simulink model "Fuel_slosh_practice"  (R2022b)
settings: Solver=FixedStepAuto  StartTime=0.0  StopTime=50.0  FixedStep=1e-3  RelTol=1e-3
values from neighbouring files (symbols this model uses):
  b = 0.1    [param.m]
  d1 = 6    [param.m]
  d2 = 10    [param.m]
  g = 9.80665    [sloshParams.m]
  k = 0.1    [param.m]
  k1 = 3    [param.m]
  k2 = 5    [param.m]
  m = 1    [param.m]
  m1 = 2    [param.m]
  m2 = 2    [param.m]
undefined symbols (not defined in the file or in its folder): L1, L2, theta1_0, theta2_0
settings Model: Creator=Aras Güngöre  LastModifiedBy=trameshk
settings SolverCC: AlgebraicLoopSolver=TrustRegion
settings DebuggingCC: UnconnectedInputMsg=warning  UnconnectedOutputMsg=warning  UnconnectedLineMsg=warning  SFMachineParentedDataDiag=warning
settings ModelReferenceCC: EnableRefExpFcnMdlSchedulingChecks=on
settings RTWCC: DLArmComputeVersion=19.05

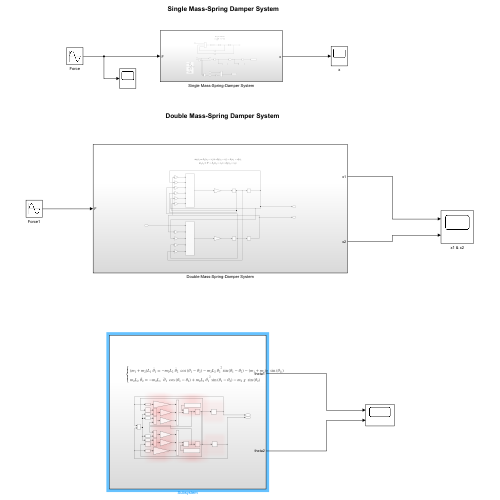
[thumbnail: Simulink's stored preview of the top-level diagram]
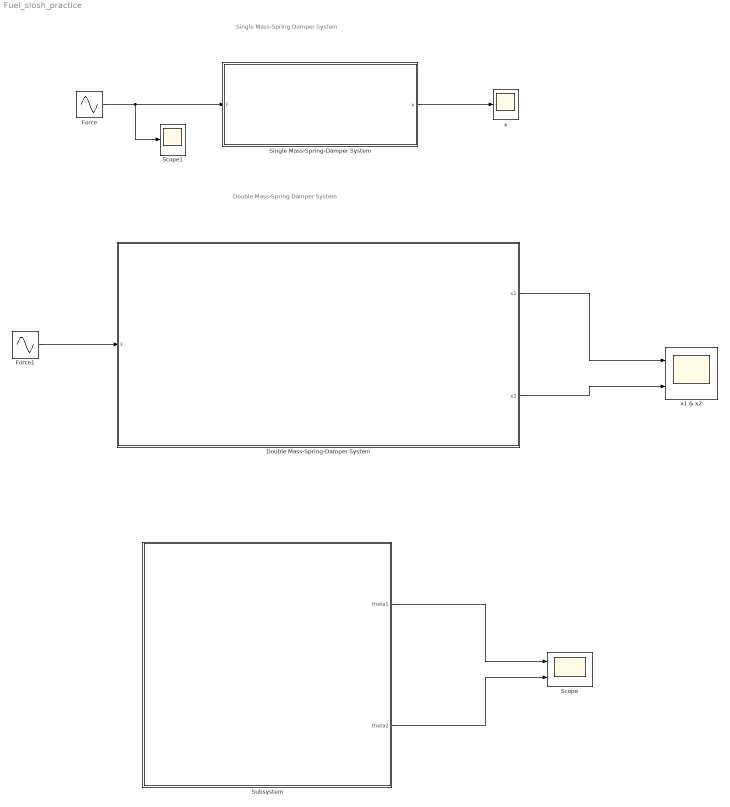
== system Fuel_slosh_practice ==
  note: Single Mass-Spring Damper System
  note: Double Mass-Spring Damper System
  Double Mass-Spring-Damper System : Subsystem
  Force : Sin  SampleTime=0
  Force1 : Sin  SampleTime=0
  Scope : Scope  NumInputPorts=2
  Scope1 : Scope
  Single Mass-Spring-Damper System : Subsystem
  Subsystem : Subsystem
  x : Scope
  x1 & x2 : Scope  NumInputPorts=2
  wires:
  Force/1 -> Scope1/1, Single Mass-Spring-Damper System/1(F)
  Single Mass-Spring-Damper System/1(x) -> x/1
  Force1/1 -> Double Mass-Spring-Damper System/1(F)
  Double Mass-Spring-Damper System/1(x1) -> x1 & x2/1
  Double Mass-Spring-Damper System/2(x2) -> x1 & x2/2
  Subsystem/2(theta2) -> Scope/2
  Subsystem/1(theta1) -> Scope/1

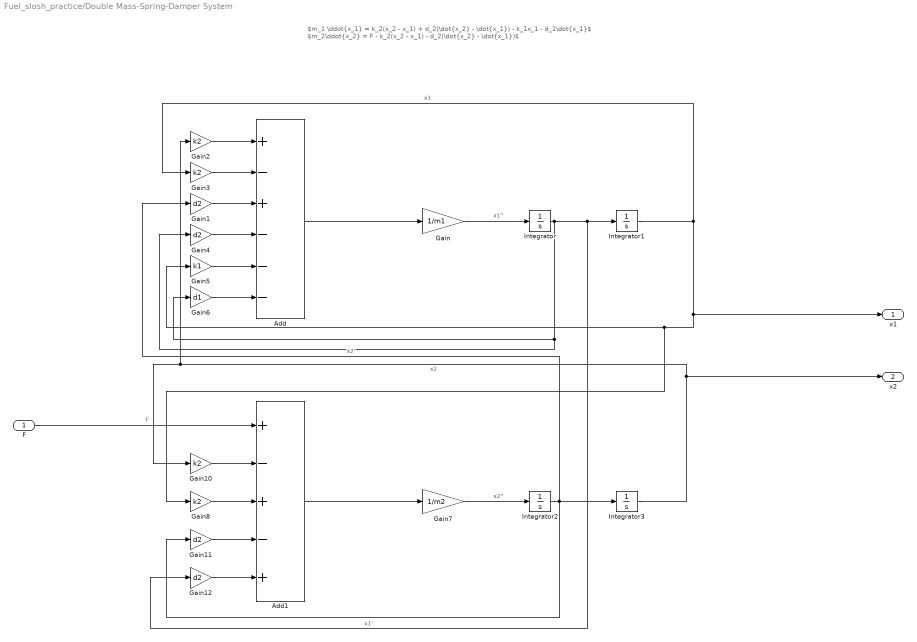
== system Fuel_slosh_practice/Double Mass-Spring-Damper System ==
  note: $m_1 \ddot{x_1} = k_2(x_2 - x_1) + d_2(\dot{x_2} - \dot{x_1}) - k_1x_1 - d_1\dot{x_1}$ $m_2\ddot{x_2} = F - k_2(x_2 - x_1) - d_2(\dot{x_2} - \dot{x_1})$
  F : Inport
  Add : Sum  Inputs=+-+---
  Add1 : Sum  Inputs=+-+-+
  Gain : Gain  Gain=1/m1
  Gain{1,4,11..12} (4 alike) : Gain  Gain=d2
  Gain{2..3,8,10} (4 alike) : Gain  Gain=k2
  Gain5 : Gain  Gain=k1
  Gain6 : Gain  Gain=d1
  Gain7 : Gain  Gain=1/m2
  Integrator{,1..3} (4 alike) : Integrator
  x1 : Outport
  x2 : Outport  Port=2
  wires:
  Integrator1/1 -> Gain3/1, x1/1, Gain8/1, Gain5/1  "x1"
  Integrator/1 -> Gain4/1, Gain6/1, Gain12/1, Integrator1/1  "x1'"
  Gain1/1 -> Add/3
  Gain3/1 -> Add/2
  Gain2/1 -> Add/1
  Add/1 -> Gain/1
  Integrator2/1 -> Gain1/1, Integrator3/1, Gain11/1  "x2'"
  Gain4/1 -> Add/4
  Gain6/1 -> Add/6
  Gain11/1 -> Add1/4
  Gain7/1 -> Integrator2/1  "x2''"
  Integrator3/1 -> x2/1, Gain10/1, Gain2/1  "x2"
  Add1/1 -> Gain7/1
  Gain10/1 -> Add1/2
  Gain5/1 -> Add/5
  Gain8/1 -> Add1/3
  Gain12/1 -> Add1/5
  Gain/1 -> Integrator/1  "x1''"
  F/1 -> Add1/1  "F"

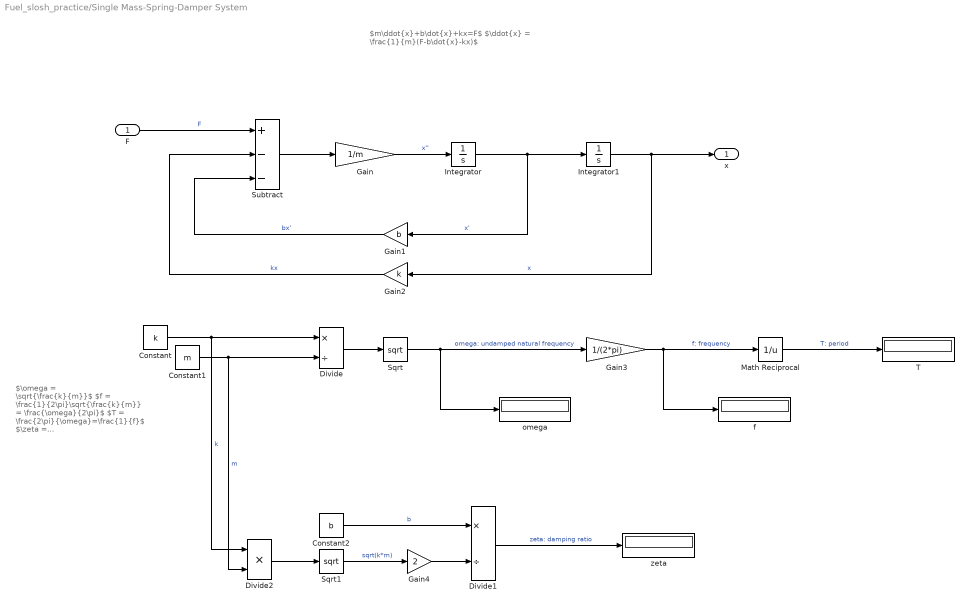
== system Fuel_slosh_practice/Single Mass-Spring-Damper System ==
  note: $\omega = \sqrt{\frac{k}{m}}$
      | $f = \frac{1}{2\pi}\sqrt{\frac{k}{m}} = \frac{\omega}{2\pi}$
      | $T = \frac{2\pi}{\omega}=\frac{1}{f}$
      | $\zeta = \frac{b}{2\sqrt{km}}$
  note: $m\ddot{x}+b\dot{x}+kx=F$
      | $\ddot{x} = \frac{1}{m}(F-b\dot{x}-kx)$
  F : Inport
  Constant : Constant  Value=k
  Constant1 : Constant  Value=m
  Constant2 : Constant  Value=b
  Divide : Product  Inputs=*/
  Divide1 : Product  Inputs=*/
  Divide2 : Product  Inputs=**
  Gain : Gain  Gain=1/m
  Gain1 : Gain  Gain=b
  Gain2 : Gain  Gain=k
  Gain3 : Gain  Gain=1/(2*pi)
  Gain4 : Gain  Gain=2
  Integrator : Integrator
  Integrator1 : Integrator
  Math Reciprocal : Math  Operator=reciprocal  SignedPower=on
  Sqrt : Sqrt
  Sqrt1 : Sqrt
  Subtract : Sum  Inputs=+--
  T : Display
  f : Display
  omega : Display
  zeta : Display
  x : Outport
  wires:
  Gain2/1 -> Subtract/2  "kx"
  Integrator1/1 -> x/1, Gain2/1  "x"
  F/1 -> Subtract/1  "F"
  Gain1/1 -> Subtract/3  "bx'"
  Integrator/1 -> Integrator1/1, Gain1/1  "x'"
  Subtract/1 -> Gain/1
  Gain/1 -> Integrator/1  "x''"
  Constant/1 -> Divide/1, Divide2/1  "k"
  Constant1/1 -> Divide2/2, Divide/2  "m"
  Divide/1 -> Sqrt/1
  Sqrt/1 -> omega/1, Gain3/1  "omega: undamped natural frequency"
  Gain3/1 -> f/1, Math Reciprocal/1  "f: frequency"
  Math Reciprocal/1 -> T/1  "T: period"
  Constant2/1 -> Divide1/1  "b"
  Sqrt1/1 -> Gain4/1  "sqrt(k*m)"
  Divide2/1 -> Sqrt1/1
  Divide1/1 -> zeta/1  "zeta: damping ratio"
  Gain4/1 -> Divide1/2

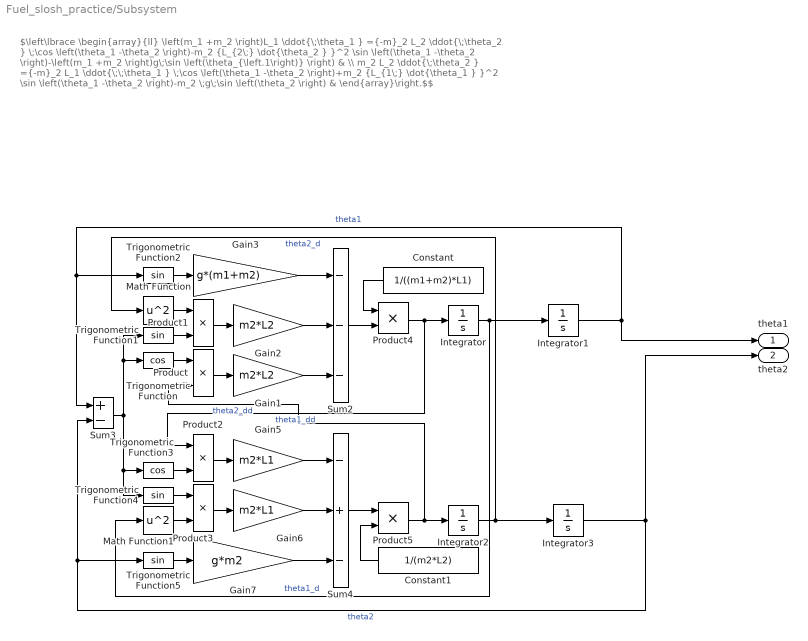
== system Fuel_slosh_practice/Subsystem ==
  note: $\left\lbrace \begin{array}{ll} \left(m_1 +m_2 \right)L_1 \ddot{\;\theta_1 } ={-m}_2 L_2 \ddot{\;\theta_2 } \;\cos \left(\theta_1 -\theta_2 \right)-m_2 {L_{2\;} \dot{\theta_2 } }^2 \sin \left(\theta_1 -\theta_2 \right)-\left(m_1 +m_2 \right)g\;\sin \left(\theta_{\left.1\right)} \right) & \\ m_2 L_2 \ddot{\;\theta_2 } ={-m}_2 L_1 \ddot{\;\;\theta_1 } \;\cos \left(\theta_1 -\theta_2 \right)+m_2 {L_{1\;} \dot{\theta_1 } }^2 \sin \left(\theta_1 -\theta_2 \right)-m_2 \;g\;\sin \left(\theta_2 \right) & \end{array}\right.$$
  Constant : Constant  Value=1/((m1+m2)*L1)  VectorParams1D=off
  Constant1 : Constant  Value=1/(m2*L2)  VectorParams1D=off
  Gain1 : Gain  Gain=m2*L2
  Gain2 : Gain  Gain=m2*L2
  Gain3 : Gain  Gain=g*(m1+m2)
  Gain5 : Gain  Gain=m2*L1
  Gain6 : Gain  Gain=m2*L1
  Gain7 : Gain  Gain=g*m2
  Integrator : Integrator  InitialCondition=[0 ]
  Integrator1 : Integrator  InitialCondition=theta1_0*pi/180
      settings: AttributesFormatString=%<InitialCondition> rad
  Integrator2 : Integrator  InitialCondition="[0  ]"
  Integrator3 : Integrator  InitialCondition=(theta2_0+theta1_0)*pi/180
      settings: AttributesFormatString=%<InitialCondition>
  Math Function : Math  Operator=square  SignedPower=on
  Math Function1 : Math  Operator=square  SignedPower=on
  Product{,1..3} (4 alike) : Product  RndMeth=Zero
  Product4 : Product
  Product5 : Product
  Sum2 : Sum  Inputs=---
  Sum3 : Sum  Inputs=+-
  Sum4 : Sum  Inputs=-+-
  Trigonometric Function : Trigonometry  Operator=cos
  Trigonometric Function{1..2,4..5} (4 alike) : Trigonometry
  Trigonometric Function3 : Trigonometry  Operator=cos
  theta1 : Outport
  theta2 : Outport  Port=2
  wires:
  Product3/1 -> Gain6/1
  Math Function1/1 -> Product3/2
  Sum4/1 -> Product5/1
  Trigonometric Function5/1 -> Gain7/1
  Trigonometric Function3/1 -> Product2/2
  Product2/1 -> Gain5/1
  Sum3/1 -> Trigonometric Function3/1, Trigonometric Function4/1, Trigonometric Function/1, Trigonometric Function1/1
  Integrator1/1 -> theta1/1, Sum3/1, Trigonometric Function2/1  "theta1"
  Product5/1 -> Integrator2/1, Product/2  "theta2_dd"
  Gain6/1 -> Sum4/2
  Integrator/1 -> Integrator1/1, Math Function1/1  "theta1_d"
  Sum2/1 -> Product4/2
  Product4/1 -> Integrator/1, Product2/1  "theta1_dd"
  Gain2/1 -> Sum2/2
  Product1/1 -> Gain2/1
  Integrator2/1 -> Math Function/1, Integrator3/1  "theta2_d"
  Integrator3/1 -> theta2/1, Trigonometric Function5/1, Sum3/2  "theta2"
  Trigonometric Function/1 -> Product/1
  Trigonometric Function1/1 -> Product1/2
  Constant/1 -> Product4/1
  Gain1/1 -> Sum2/3
  Constant1/1 -> Product5/2
  Trigonometric Function2/1 -> Gain3/1
  Gain5/1 -> Sum4/1
  Trigonometric Function4/1 -> Product3/1
  Gain7/1 -> Sum4/3
  Gain3/1 -> Sum2/1
  Math Function/1 -> Product1/1
  Product/1 -> Gain1/1
